simulink model "quarter_sus_imp"  (R2025a)
settings: Solver=FixedStepAuto  StartTime=0.0  StopTime=20  FixedStep=0.001  RelTol=1e-3
model workspace (MAT data in the model file):
  Cs = Simulink.Parameter
  Cs.Value = 2000
  Cs.Complexity = 'real'
  Cs.Dimensions = [1 1]
  Cs.DataType = 'auto'
  Cy_f1 = 128915.5
  Cy_r1 = 85943.6
  G0 = Simulink.Parameter
  G0.Value = 0.000256
  G0.Complexity = 'real'
  G0.Dimensions = [1 1]
  G0.DataType = 'auto'
  IDA_ISD_PBC_bd = Simulink.Parameter
  IDA_ISD_PBC_bd.Value = 300
  IDA_ISD_PBC_bd.Complexity = 'real'
  IDA_ISD_PBC_bd.Dimensions = [1 1]
  IDA_ISD_PBC_bd.DataType = 'auto'
  IDA_ISD_PBC_c1 = Simulink.Parameter
  IDA_ISD_PBC_c1.Value = 1500
  IDA_ISD_PBC_c1.Complexity = 'real'
  IDA_ISD_PBC_c1.Dimensions = [1 1]
  IDA_ISD_PBC_c1.DataType = 'auto'
  IDA_ISD_PBC_k1 = Simulink.Parameter
  IDA_ISD_PBC_k1.Value = 10000
  IDA_ISD_PBC_k1.Complexity = 'real'
  IDA_ISD_PBC_k1.Dimensions = [1 1]
  IDA_ISD_PBC_k1.DataType = 'auto'
  IDA_ISD_PBC_k2 = Simulink.Parameter
  IDA_ISD_PBC_k2.Value = 5000
  IDA_ISD_PBC_k2.Complexity = 'real'
  IDA_ISD_PBC_k2.Dimensions = [1 1]
  IDA_ISD_PBC_k2.DataType = 'auto'
  IDA_ISD_PBC_r1 = Simulink.Parameter
  IDA_ISD_PBC_r1.Value = 1
  IDA_ISD_PBC_r1.Complexity = 'real'
  IDA_ISD_PBC_r1.Dimensions = [1 1]
  IDA_ISD_PBC_r1.DataType = 'auto'
  IDA_PBC_cd4 = 2000
  IDA_PBC_kd2 = 10000
  IDA_PBC_r1 = 1.5
  IDA_PBC_r2 = 0.44
  ISD_1_b = Simulink.Parameter
  ISD_1_b.Value = 158
  ISD_1_b.Complexity = 'real'
  ISD_1_b.Dimensions = [1 1]
  ISD_1_b.DataType = 'auto'
  ISD_1_c = Simulink.Parameter
  ISD_1_c.Value = 500
  ISD_1_c.Complexity = 'real'
  ISD_1_c.Dimensions = [1 1]
  ISD_1_c.DataType = 'auto'
  ISD_1_k1 = Simulink.Parameter
  ISD_1_k1.Value = 1000
  ISD_1_k1.Complexity = 'real'
  ISD_1_k1.Dimensions = [1 1]
  ISD_1_k1.DataType = 'auto'
  ISD_1_k2 = Simulink.Parameter
  ISD_1_k2.Value = 1000
  ISD_1_k2.Complexity = 'real'
  ISD_1_k2.Dimensions = [1 1]
  ISD_1_k2.DataType = 'auto'
  Izz1 = 1536.7
  Ks = Simulink.Parameter
  Ks.Value = 20000
  Ks.Complexity = 'real'
  Ks.Dimensions = [1 1]
  Ks.DataType = 'auto'
  Kt = Simulink.Parameter
  Kt.Value = 200000
  Kt.Complexity = 'real'
  Kt.Dimensions = [1 1]
  Kt.DataType = 'auto'
  Q = Simulink.Parameter
  Q.Value = [0.1  0  0  0; 0  0.1  0  0; 0  0  1  0; 0  0  0  0.1]
  Q.Complexity = 'real'
  Q.Dimensions = [4 4]
  Q.DataType = 'auto'
  Q_dot = Simulink.Parameter
  Q_dot.Value = [1  0; 0  0.001]
  Q_dot.Complexity = 'real'
  Q_dot.Dimensions = [2 2]
  Q_dot.DataType = 'auto'
  Q_dot_s = Simulink.Parameter
  Q_dot_s.Value = 1
  Q_dot_s.Complexity = 'real'
  Q_dot_s.Dimensions = [1 1]
  Q_dot_s.DataType = 'auto'
  Q_dot_u = Simulink.Parameter
  Q_dot_u.Value = 0.001
  Q_dot_u.Complexity = 'real'
  Q_dot_u.Dimensions = [1 1]
  Q_dot_u.DataType = 'auto'
  Q_flec = Simulink.Parameter
  Q_flec.Value = 2.5
  Q_flec.Complexity = 'real'
  Q_flec.Dimensions = [1 1]
  Q_flec.DataType = 'auto'
  SHADD_alpha = Simulink.Parameter
  SHADD_alpha.Value = 11.9
  SHADD_alpha.Complexity = 'real'
  SHADD_alpha.Dimensions = [1 1]
  SHADD_alpha.DataType = 'auto'
  a1 = 1.015
  a_max = Simulink.Parameter
  a_max.Value = 4000
  a_max.Complexity = 'real'
  a_max.Dimensions = [1 1]
  a_max.DataType = 'auto'
  a_min = Simulink.Parameter
  a_min.Value = -4000
  a_min.Complexity = 'real'
  a_min.Dimensions = [1 1]
  a_min.DataType = 'auto'
  adva_max = Simulink.Parameter
  adva_max.Value = 300
  adva_max.Complexity = 'real'
  adva_max.Dimensions = [1 1]
  adva_max.DataType = 'auto'
  adva_min = Simulink.Parameter
  adva_min.Value = -300
  adva_min.Complexity = 'real'
  adva_min.Dimensions = [1 1]
  adva_min.DataType = 'auto'
  as_max = Simulink.Parameter
  as_max.Value = 2
  as_max.Complexity = 'real'
  as_max.Dimensions = [1 1]
  as_max.DataType = 'auto'
  b1 = 1.895
  b_deflec = Simulink.Parameter
  b_deflec.Value = 0.04
  b_deflec.Complexity = 'real'
  b_deflec.Dimensions = [1 1]
  b_deflec.DataType = 'auto'
  b_deflec.DocUnits = 'm'
  bump_height = Simulink.Parameter
  bump_height.Value = 0.02
  bump_height.Complexity = 'real'
  bump_height.Dimensions = [1 1]
  bump_height.DataType = 'auto'
  bump_lenth = Simulink.Parameter
  bump_lenth.Value = 0.3
  bump_lenth.Complexity = 'real'
  bump_lenth.Dimensions = [1 1]
  bump_lenth.DataType = 'auto'
  bump_start = Simulink.Parameter
  bump_start.Value = 1
  bump_start.Complexity = 'real'
  bump_start.Dimensions = [1 1]
  bump_start.DataType = 'auto'
  damper_param = Simulink.Parameter
  damper_param.Value = [-3991.04201041 6552.27356799 -1014.47680093 15090.2668269 -24778.0492645 8455.72459788 2073.28613088 -842.442698484 15.8288582111 -42.6273340405 228.645778088 77.1011895387 -307.938386665 98.5439708573 7.35255277487 0.432771680092]
  damper_param.Complexity = 'real'
  damper_param.Dimensions = [1 16]
  damper_param.DataType = 'auto'
  deflec_max = Simulink.Parameter
  deflec_max.Value = 0.02
  deflec_max.Complexity = 'real'
  deflec_max.Dimensions = [1 1]
  deflec_max.DataType = 'auto'
  done_range = Simulink.Parameter
  done_range.Value = [6 5 0.523598775598]
  done_range.Complexity = 'real'
  done_range.Dimensions = [1 3]
  done_range.DataType = 'double'
  f0 = Simulink.Parameter
  f0.Value = 0.1
  f0.Complexity = 'real'
  f0.Dimensions = [1 1]
  f0.DataType = 'auto'
  h1 = 0.54
  imp_Cs = Simulink.Parameter
  imp_Cs.Value = 1800
  imp_Cs.Complexity = 'real'
  imp_Cs.Dimensions = [1 1]
  imp_Cs.DataType = 'auto'
  imp_Ks = Simulink.Parameter
  imp_Ks.Value = 20500
  imp_Ks.Complexity = 'real'
  imp_Ks.Dimensions = [1 1]
  imp_Ks.DataType = 'auto'
  imp_Ms = Simulink.Parameter
  imp_Ms.Value = 370
  imp_Ms.Complexity = 'real'
  imp_Ms.Dimensions = [1 1]
  imp_Ms.DataType = 'auto'
  inerter_b = Simulink.Parameter
  inerter_b.Value = 300
  inerter_b.Complexity = 'real'
  inerter_b.Dimensions = [1 1]
  inerter_b.DataType = 'auto'
  inerter_b_2 = Simulink.Parameter
  inerter_b_2.Value = 2
  inerter_b_2.Complexity = 'real'
  inerter_b_2.Dimensions = [1 1]
  inerter_b_2.DataType = 'auto'
  inerter_c = Simulink.Parameter
  inerter_c.Value = 2000
  inerter_c.Complexity = 'real'
  inerter_c.Dimensions = [1 1]
  inerter_c.DataType = 'auto'
  inerter_k = Simulink.Parameter
  inerter_k.Value = 5000
  inerter_k.Complexity = 'real'
  inerter_k.Dimensions = [1 1]
  inerter_k.DataType = 'auto'
  inerter_k_2 = Simulink.Parameter
  inerter_k_2.Value = 10000
  inerter_k_2.Complexity = 'real'
  inerter_k_2.Dimensions = [1 1]
  inerter_k_2.DataType = 'auto'
  ms = Simulink.Parameter
  ms.Value = 400
  ms.Complexity = 'real'
  ms.Dimensions = [1 1]
  ms.DataType = 'auto'
  mu = Simulink.Parameter
  mu.Value = 40
  mu.Complexity = 'real'
  mu.Dimensions = [1 1]
  mu.DataType = 'auto'
  noise_seed = Simulink.Parameter
  noise_seed.Value = 23341
  noise_seed.Complexity = 'real'
  noise_seed.Dimensions = [1 1]
  noise_seed.DataType = 'auto'
  punish_Q = Simulink.Parameter
  punish_Q.Value = [10 0.1 1]
  punish_Q.Complexity = 'real'
  punish_Q.Dimensions = [1 3]
  punish_Q.DataType = 'auto'
  punish_R = Simulink.Parameter
  punish_R.Value = 0
  punish_R.Complexity = 'real'
  punish_R.Dimensions = [1 1]
  punish_R.DataType = 'auto'
  reward_w_as = Simulink.Parameter
  reward_w_as.Value = 2
  reward_w_as.Complexity = 'real'
  reward_w_as.Dimensions = [1 1]
  reward_w_as.DataType = 'auto'
  reward_w_au = Simulink.Parameter
  reward_w_au.Value = 40
  reward_w_au.Complexity = 'real'
  reward_w_au.Dimensions = [1 1]
  reward_w_au.DataType = 'auto'
  reward_w_defv = Simulink.Parameter
  reward_w_defv.Value = 0.6
  reward_w_defv.Complexity = 'real'
  reward_w_defv.Dimensions = [1 1]
  reward_w_defv.DataType = 'auto'
  road_seed = Simulink.Parameter
  road_seed.Value = 9759
  road_seed.Complexity = 'real'
  road_seed.Dimensions = [1 1]
  road_seed.DataType = 'auto'
  road_type = Simulink.Parameter
  road_type.Value = 3
  road_type.Complexity = 'real'
  road_type.Dimensions = [1 1]
  road_type.DataType = 'int8'
  sigma_f1 = 0.1
  sigma_r1 = 0.1
  sine_amp = Simulink.Parameter
  sine_amp.Value = 0.01
  sine_amp.Complexity = 'real'
  sine_amp.Dimensions = [1 1]
  sine_amp.DataType = 'auto'
  sine_amp.DocUnits = 'm'
  sine_freq = Simulink.Parameter
  sine_freq.Value = 4
  sine_freq.Complexity = 'real'
  sine_freq.Dimensions = [1 1]
  sine_freq.DataType = 'auto'
  sine_freq.DocUnits = 'Hz'
  u = Simulink.Parameter
  u.Value = 22.2222
  u.Complexity = 'real'
  u.Dimensions = [1 1]
  u.DataType = 'auto'
  vs0 = Simulink.Parameter
  vs0.Value = 0
  vs0.Complexity = 'real'
  vs0.Dimensions = [1 1]
  vs0.DataType = 'auto'
  vu0 = Simulink.Parameter
  vu0.Value = 0
  vu0.Complexity = 'real'
  vu0.Dimensions = [1 1]
  vu0.DataType = 'auto'
  x_max = Simulink.Parameter
  x_max.Value = [9999 9999 9999 9999 9999 9999 9999 9999 9999 9999 9999 9999]
  x_max.Complexity = 'real'
  x_max.Dimensions = [1 12]
  x_max.DataType = 'auto'
  x_min = Simulink.Parameter
  x_min.Value = [-9999 -9999 -9999 -9999 -9999 -9999 -9999 -9999 -9999 -9999 -9999 9999]
  x_min.Complexity = 'real'
  x_min.Dimensions = [1 12]
  x_min.DataType = 'auto'
  xs0 = Simulink.Parameter
  xs0.Value = 0
  xs0.Complexity = 'real'
  xs0.Dimensions = [1 1]
  xs0.DataType = 'auto'
  xu0 = Simulink.Parameter
  xu0.Value = 0
  xu0.Complexity = 'real'
  xu0.Dimensions = [1 1]
  xu0.DataType = 'auto'
undefined symbols (not defined in the file or in its folder): ADD, Force, IDA, Imp, PBC, SH, Train, Validation
libraries: fl_lib x32, nesl_utility x27, sdl_lib x2, deeplib x1, simulink x1
(part 1 of 5)
settings Model: PauseTimes=3  TunableVars=a_max,a_min,adva_max,adva_min,x_ini,x_max,x_min  TunableVarsStorageClass=Auto,Auto,Auto,Auto,Auto,Auto,Auto  TunableVarsTypeQualifier=,,,,,,  ParameterArgumentNames=Cs,G0,Ks,Kt,Q,Q_dot,Q_dot_s,Q_dot_u,Q_flec,a_max,a_min,adva_max,adva_min,as_max,b_deflec,bump_height,bump_lenth,bump_start,damper_param,deflec_max,done_range,f0,inerter_b,inerter_b_2,inerter_c,inerter_k,inerter_k_2,ms,mu,noise_seed,punish_Q,punish_R,road_seed,road_type,sine_amp,sine_freq,u,vs0,vu0,x_max,x_min,xs0,xu0  Creator=hjzsj  LastModifiedBy=Asus
settings ConfigSet: Description=Config for code generation python binding.
settings OptimizationCC: DefaultParameterBehavior=Inlined  UseDivisionForNetSlopeComputation=on  UseFloatMulNetSlope=on  StrengthReduction=on  PassReuseOutputArgsAs=Individual arguments  ZeroExternalMemoryAtStartup=off  ZeroInternalMemoryAtStartup=off  NoFixptDivByZeroProtection=on  EfficientFloat2IntCast=on  OptimizeBlockOrder=speed  OptimizationPriority=Speed  OptimizationCustomize=off  MultiThreadedLoops=on  AutoScheduleForLoops=on  EfficientTunableParamExpr=on
settings DebuggingCC: ParameterTunabilityLossMsg=error  UnconnectedInputMsg=warning  UnconnectedOutputMsg=warning  UnconnectedLineMsg=warning  ArithmeticOperatorsInVariantConditions=warning
settings HardwareCC: ProdLongLongMode=on  TargetPreprocMaxBitsSint=64.0  TargetPreprocMaxBitsUint=64.0
settings ModelReferenceCC: EnableRefExpFcnMdlSchedulingChecks=on
settings SFSimCC: MATLABDynamicMemAlloc=off  CustomCodeUndefinedFunction=UseInterfaceOnly  SimTargetLang=C++  SimDLTargetLibrary=mkl-dnn
settings RTWCC: SystemTargetFile=ert.tlc  GenCodeOnly=on  TemplateMakefile=ert_default_tmf  PostCodeGenCommand=slxpy.postprocess(modelName,buildInfo)  RetainRTWFile=on  Toolchain=MinGW64 | gmake (64-bit Windows)  BuildConfiguration=Debug  PortableWordSizes=on  TargetLang=C++  GPUComputeCapability=3.5  DLArmComputeVersion=19.05  Description=Embedded Coder
settings CodeAppCC: ForceParamTrailComments=on  CommentStyle=Multi-line  IgnoreCustomStorageClasses=off  MaxIdLength=64.0  OperatorAnnotations=on  SimulinkDataObjDesc=on  SFDataObjDesc=on  MATLABFcnDesc=on  MangleLength=4.0  InsertBlockDesc=on  StateflowObjectComments=on  MATLABSourceComments=on
settings ERTTargetCC: ExtModeTransport=0.0  ExtModeStaticAlloc=off  ExtModeMexFile=ext_comm  ExtModeIntrfLevel=Level1  RootIOFormat=Structure reference  ERTCustomFileTemplate=example_file_process.tlc  TargetLangStandard=C++11 (ISO)  CodeInterfacePackaging=C++ class  SubcomponentCodeInterfacePackaging=C++ class  SupportComplex=off  SupportContinuousTime=on  SupportVariableSizeSignals=on

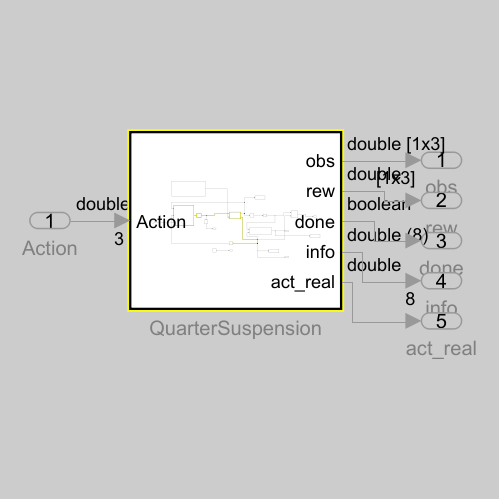
[thumbnail: Simulink's stored preview of the top-level diagram]
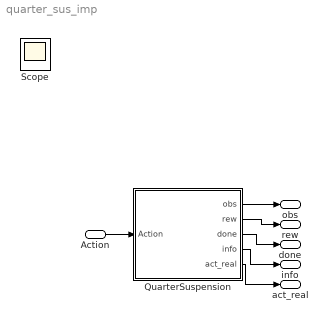
== system quarter_sus_imp ==
  Action : Inport  PortDimensions=3
  "QuarterSuspension " : Subsystem
  obs : Outport
  rew : Outport  Port=2
  done : Outport  Port=3
  info : Outport  Port=4
  act_real : Outport  Port=5
  Scope : Scope
      settings: ActiveDisplayYMinimum=-0.0848  ActiveDisplayYMaximum=0.15745
  wires:
  "QuarterSuspension "/1(obs) -> obs/1
  "QuarterSuspension "/2(rew) -> rew/1
  Action/1 -> "QuarterSuspension "/1(Action)
  "QuarterSuspension "/3(done) -> done/1
  "QuarterSuspension "/4(info) -> info/1
  "QuarterSuspension "/5(act_real) -> act_real/1

== system quarter_sus_imp/QuarterSuspension  ==
  Action : Inport
  Constant : Constant  Value=0  OutDataTypeStr=boolean
  Memory : Memory
  Reshape : Reshape  OutputDimensionality=Row vector (2-D)
  Saturation2 : Saturate  UpperLimit=a_max  LowerLimit=a_min
  Subsystem1 : Subsystem  Variant=on  VariantControlMode=label  VariantControl=Choice  LabelModeActiveChoice=Semi-active Air
  To Workspace : ToWorkspace  VariableName=state  SampleTime=-1
  To Workspace1 : ToWorkspace  VariableName=reward  SampleTime=-1
  To Workspace2 : ToWorkspace  VariableName=info  SampleTime=-1
  Variant Subsystem : Subsystem  Variant=on  VariantControlMode=label  LabelModeActiveChoice=Train-Imp
  Zero-Order Hold : ZeroOrderHold  SampleTime=-1
  Zero-Order Hold2 : ZeroOrderHold  SampleTime=-1
  obs_route : Subsystem
  reward_cal : Subsystem
  road_profile : Subsystem  Variant=on  VariantControlMode=label  LabelModeActiveChoice=OriginRoad
  obs : Outport
  rew : Outport  Port=2
  done : Outport  Port=3
  info : Outport  Port=4
  act_real : Outport  Port=5
  wires:
  Action/1 -> Variant Subsystem/3(train_action)
  Zero-Order Hold/1 -> Reshape/1
  Reshape/1 -> reward_cal/1(state), obs_route/1(state)
  Subsystem1/2(info) -> reward_cal/2(info), To Workspace2/1, info/1, Memory/1, obs_route/2(In3)
  Constant/1 -> done/1
  Variant Subsystem/1(action) -> Saturation2/1
  Saturation2/1 -> Zero-Order Hold2/1, Subsystem1/1(act)
  Zero-Order Hold2/1 -> act_real/1
  road_profile/1("Road ") -> Subsystem1/2(xr)
  Subsystem1/1(state) -> Variant Subsystem/1(state), To Workspace/1, Zero-Order Hold/1
  obs_route/1(obs_out) -> obs/1
  reward_cal/1(reward) -> rew/1, To Workspace1/1
  Memory/1 -> Variant Subsystem/2(ref_info)

== system quarter_sus_imp/QuarterSuspension /Subsystem1 ==
  act : Inport
  xr : Inport  Port=2
  Active Suspension : Subsystem  VariantControl=Active
  Semi Active Air Suspension : Subsystem  VariantControl=Semi-active Air
  Semi Active Air Suspension simscape : Subsystem  VariantControl=Semi-active Air Simscape
  Semi Active Suspension : Subsystem  VariantControl=Semi-active
  state : Outport
  info : Outport  Port=2

== system quarter_sus_imp/QuarterSuspension /Variant Subsystem ==
  note: 1) Add Subsystem or Model blocks as valid variant choices.
      | 2) You cannot connect blocks at this level. At simulation, connectivity is automatically
      | determined, based on the active variant and port name matching.
  state : Inport
  ref_info : Inport  Port=2
  train_action : Inport  Port=3  PortDimensions=3
  ADD : Subsystem  VariantControl=ADD
  H1_power_min : Subsystem  VariantControl=H1_Power_min
  IDA-PBC : Subsystem  VariantControl=IDA-PBC
  Openloop : Subsystem  VariantControl=Opneloop
  PDD : Subsystem  VariantControl=PDD
  SH-ADD : Subsystem  VariantControl=SH-ADD
  Skyhook : Subsystem  VariantControl=SkyHook
  Train-Force : Subsystem  VariantControl=Train-Force
  Train-Imp : Subsystem  VariantControl=Train-Imp
  Vaildation-3para-feedback : Subsystem  VariantControl=Validation-3para-back
  Vaildation-Force : Subsystem  VariantControl=Validation-Force
  Vaildation-Imp : Subsystem  VariantControl=Validation-Imp
  impedance : Subsystem  VariantControl=Impedance
  train_IMP_force : Subsystem  VariantControl=Subsystem
  action : Outport

== system quarter_sus_imp/QuarterSuspension /obs_route ==
  state : Inport
  In3 : Inport  Port=2
  Add : Sum  Inputs=+-
  Reshape : Reshape  OutputDimensionality=Row vector (2-D)
  Selector : Selector  InputPortWidth=8  IndexOptions=Index vector (dialog)  Indices=[7 8]  OutputSizes=1
  Selector1 : Selector  InputPortWidth=4  IndexOptions=Index vector (dialog)  Indices=[1]  OutputSizes=1
  Selector2 : Selector  InputPortWidth=4  IndexOptions=Index vector (dialog)  Indices=[3]  OutputSizes=1
  Vector Concatenate : Concatenate
  obs_out : Outport
  wires:
  Selector/1 -> Vector Concatenate/2
  Selector2/1 -> Add/2
  In3/1 -> Selector/1
  state/1 -> Selector2/1, Selector1/1
  Vector Concatenate/1 -> Reshape/1
  Selector1/1 -> Add/1
  Add/1 -> Vector Concatenate/1
  Reshape/1 -> obs_out/1

== system quarter_sus_imp/QuarterSuspension /reward_cal ==
  state : Inport
  info : Inport  Port=2
  Add : Sum
  Add1 : Sum  Inputs=+-
  Add2 : Sum
  Constant1 : Constant  Value=Q_flec
  Constant3 : Constant  Value=b_deflec
  Demux : Demux  Outputs=2
  Gain : Gain  Gain=Q_dot_s
  Gain1 : Gain  Gain=Q_dot_u
  Gain2 : Gain  Gain=-1
  Selector : Selector  InputPortWidth=8  IndexOptions=Index vector (dialog)  Indices=[7 8]  OutputSizes=1
  Selector1 : Selector  InputPortWidth=4  IndexOptions=Index vector (dialog)  Indices=[1]  OutputSizes=1
  Selector2 : Selector  InputPortWidth=4  IndexOptions=Index vector (dialog)  Indices=[3]  OutputSizes=1
  Square : Math  Operator=square
  Square1 : Math  Operator=square
  cal_reward : MATLAB Function  TreatAsAtomicUnit=on
  reward : Outport
  wires:
  Constant1/1 -> cal_reward/3(Q_flec)
  Constant3/1 -> cal_reward/2(b_def)
  cal_reward/1(reward) -> Add/1  "reward_deflec"
  Add/1 -> Gain2/1  "reward"
  Add2/1 -> Add/2  "reward_dot"
  state/1 -> Selector2/1, Selector1/1
  Selector2/1 -> Add1/2
  Selector1/1 -> Add1/1
  Add1/1 -> cal_reward/1(state_deflec)
  info/1 -> Selector/1
  Selector/1 -> Demux/1
  Demux/1 -> Square/1
  Demux/2 -> Square1/1
  Square/1 -> Gain/1
  Square1/1 -> Gain1/1
  Gain2/1 -> reward/1
  Gain/1 -> Add2/1  "reward_accs"
  Gain1/1 -> Add2/2  "reward_accu"

== system quarter_sus_imp/QuarterSuspension /road_profile ==
  note: 1) Add Subsystem or Model blocks as valid variant choices.
      | 2) You cannot connect blocks at this level. At simulation, connectivity is automatically
      | determined, based on the active variant and port name matching.
  Subsystem : Subsystem  VariantControl=Look table
  gp : Subsystem  VariantControl=GpSample
  origin : Subsystem  VariantControl=OriginRoad
  "Road " : Outport

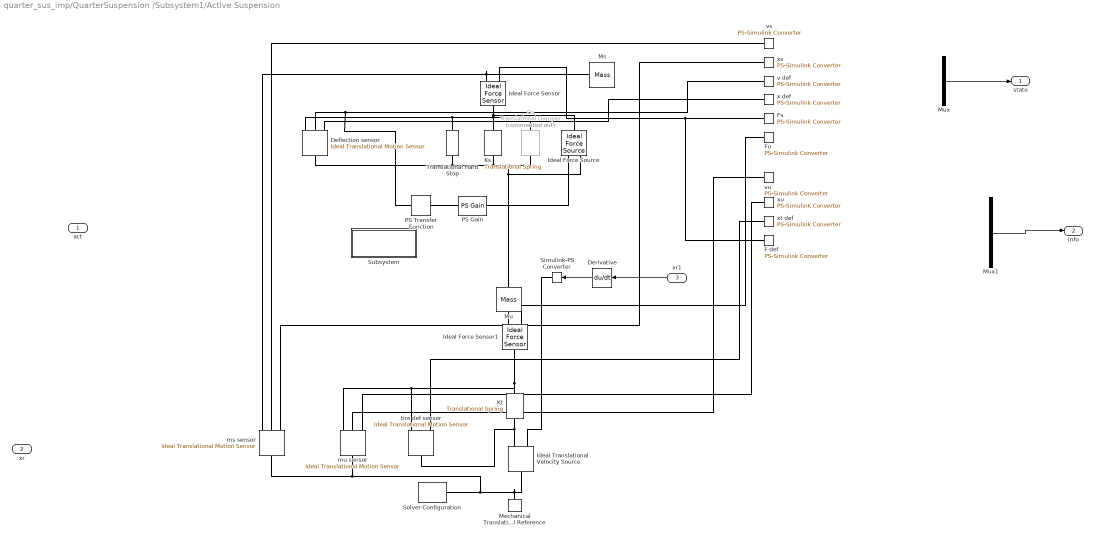
== system quarter_sus_imp/QuarterSuspension /Subsystem1/Active Suspension ==
  act : Inport
  xr : Inport  Port=2
  xr1 : Inport  Port=3
  Cs : fl_lib/Mechanical/Translational Elements/Translational Damper  Commented=on  D=2000 N*s/m  v_specify=on  v_priority=None  v=0 m/s  v_nominal_specify=off  v_nominal_unit=m/s  v_nominal_value=1  f_specify=off  f_priority=None  f=0 N  f_nominal_specify=off  f_nominal_unit=N  f_nominal_value=1
  Deflection sensor : fl_lib/Mechanical/Mechanical Sensors/Ideal Translational Motion Sensor  reference=foundation.enum.MeasurementReference.difference  acceleration_port=false  velocity_port=true  position_port=true  offset=0 m
  Derivative : Derivative
  F def : nesl_utility/PS-Simulink Converter  PhysicalDomain=network_engine_domain  SubClassName=ps_output  LeftPortType=input  RightPortType=output  PseudoPeriodic=off  Frequencies=[]  VectorFormat=inherit  Unit=inherit  AffineConversion=off
  Fs : nesl_utility/PS-Simulink Converter  PhysicalDomain=network_engine_domain  SubClassName=ps_output  LeftPortType=input  RightPortType=output  PseudoPeriodic=off  Frequencies=[]  VectorFormat=inherit  Unit=inherit  AffineConversion=off
  Fu : nesl_utility/PS-Simulink Converter  PhysicalDomain=network_engine_domain  SubClassName=ps_output  LeftPortType=input  RightPortType=output  PseudoPeriodic=off  Frequencies=[]  VectorFormat=inherit  Unit=inherit  AffineConversion=off
  Ideal Force Sensor : fl_lib/Mechanical/Mechanical Sensors/Ideal Force Sensor
  Ideal Force Sensor1 : fl_lib/Mechanical/Mechanical Sensors/Ideal Force Sensor
  Ideal Force Source : fl_lib/Mechanical/Mechanical Sources/Ideal Force Source
      settings: LogSimulationData=on
  Ideal Translational Velocity Source : fl_lib/Mechanical/Mechanical Sources/Ideal Translational Velocity Source
  Ks : fl_lib/Mechanical/Translational Elements/Translational Spring  spr_rate=20000 N/m  v_specify=off  v_priority=None  v=0 m/s  v_nominal_specify=off  v_nominal_unit=m/s  v_nominal_value=1  f_specify=off  f_priority=None  f=0 N  f_nominal_specify=off  f_nominal_unit=N  f_nominal_value=1  x_specify=on  x_priority=High  x=0 m  x_nominal_specify=off  x_nominal_unit=m  x_nominal_value=1
  Kt : fl_lib/Mechanical/Translational Elements/Translational Spring  spr_rate=200000 N/m  v_specify=off  v_priority=None  v=0 m/s  v_nominal_specify=off  v_nominal_unit=m/s  v_nominal_value=1  f_specify=off  f_priority=None  f=0 N  f_nominal_specify=off  f_nominal_unit=N  f_nominal_value=1  x_specify=on  x_priority=High  x=0 m  x_nominal_specify=off  x_nominal_unit=m  x_nominal_value=1
  Mechanical Translational Reference : fl_lib/Mechanical/Translational Elements/Mechanical Translational Reference
  Ms : fl_lib/Mechanical/Translational Elements/Mass  mass=400 kg  num_ports=foundation.enum.numPorts2.one  v_specify=off  v_priority=High  v=0 m/s  v_nominal_specify=off  v_nominal_unit=m/s  v_nominal_value=1  f_specify=off  f_priority=None  f=0 N  f_nominal_specify=off  f_nominal_unit=N  f_nominal_value=1
  Mu : fl_lib/Mechanical/Translational Elements/Mass  mass=40 kg  num_ports=foundation.enum.numPorts2.two  v_specify=off  v_priority=High  v=0 m/s  v_nominal_specify=off  v_nominal_unit=m/s  v_nominal_value=1  f_specify=off  f_priority=None  f=0 N  f_nominal_specify=off  f_nominal_unit=N  f_nominal_value=1
      settings: InternalSimscapePortConfiguration="{\"Bottom\":[],\"Left\":[{\"id\":\"M\",\"label\":\"\",\"type\":\"foundation.mechanical.translational.translational\"}],\"Right\":[{\"id\":\"N\",\"label\":\"\",\"type\":\"foundation.mechanical.translational.translational\"}],\"Top\":[]}"
  Mux : Mux
  Mux1 : Mux  Inputs=8
  PS Gain : fl_lib/Physical Signals/Functions/PS Gain  gain=2000 N*s/m
  PS Transfer Function : fl_lib/Physical Signals/Linear Operators/PS Transfer Function  transfer_function_type=foundation.enum.transfer_function_type.lag  T=20 ms  T1=2 s  T2=1 s  reset_method=foundation.enum.IntegratorResetSpec.None  initial_condition_spec=foundation.enum.IntegratorICSpec.Internal  y0=0 m/s
      settings: InternalSimscapePortConfiguration="{\"Bottom\":[],\"Left\":[{\"id\":\"U\",\"label\":\"\",\"type\":\"input\"}],\"Right\":[{\"id\":\"Y\",\"label\":\"\",\"type\":\"output\"}],\"Top\":[]}"
  Simulink-PS Converter : nesl_utility/Simulink-PS Converter  PhysicalDomain=network_engine_domain  SubClassName=ps_input  LeftPortType=input  RightPortType=output  PseudoPeriodic=off  Frequencies=[]  NoiseDistribution=none  NoiseParameters=[]  Unit=1  AffineConversion=off  FilteringAndDerivatives=provide  SimscapeFilterOrder=1  InputFilterTimeConstant=0.001  UdotUserProvided=0
  Solver Configuration : nesl_utility/Solver Configuration  PhysicalDomain=network_engine_domain  SubClassName=solver  LeftPortType=input  RightPortType=generic  Tones=[]  Harmonics=[]  SimulateNoise=off  Profile=off  UseLocalSampling=off  EnableSwitchedLinearOptims=on  FrequencyDomain=off  UseCCode=off  RelTol=0.001  AbsTol=1e-06  MinStep=1e-09  ToWorkspace=off  RevertToSquareIcSolve=off  NumHomotopyIterations=100  PhasorMode=off  PhasorModeNumHarmonics=1  ConsistencySolver=NEWTON_XTOL_AFTER_FTOL  IndexReductionMethod=DerivativeReplacement  DoDC=off  ResidualTolerance=1e-09  ConsistencyTolSource=GLOBAL  ConsistencyAbsTol=0.001  ConsistencyRelTol=0.001  ConsistencyTolFactor=0.001  UseLocalSolver=off  LocalSolverChoice=NE_BACKWARD_EULER_ADVANCER  ResolveIndetEquations=on  FunctionEvalNumThread=1  LocalSolverSampleTime=0.001  DoFixedCost=off  MaxNonlinIter=3  MaxModeIter=2  ComputeImpulses=off  ImpulseIterations=2  LinearAlgebra=auto  LinearAlgebraNumThread=0  EquationFormulation=NE_TIME_EF  DelaysMemoryBudget=1024  AutomaticFiltering=on  FilteringTimeConstant=0.001  PartitionStorageMethod=AS_NEEDED  PartitionMemoryBudget=1024  PartitionMethod=ROBUST
  Subsystem : Subsystem
  Translational Hard Stop : fl_lib/Mechanical/Translational Elements/Translational Hard Stop  upper_bnd=0.2 m  lower_bnd=-0.2 m  model=simscape.enum.hardstop.smooth  stiff_up=1e6 N/m  stiff_low=1e6 N/m  D_up=150 N*s/m  D_low=150 N*s/m  transition=0.01 mm  coeff_rest=0.7  v_tol=0.001 m/s  f_tol=0.001 N  x_specify=on  x_priority=High  x=0 m  x_nominal_specify=off  x_nominal_unit=m  x_nominal_value=1  v_specify=off  v_priority=None  v=0 m/s  v_nominal_specify=off  v_nominal_unit=m/s  v_nominal_value=1  f_specify=off  f_priority=None  f=0 N  f_nominal_specify=off  f_nominal_unit=N  f_nominal_value=1  M_specify=off  M_priority=None  M=0
  ms sensor : fl_lib/Mechanical/Mechanical Sensors/Ideal Translational Motion Sensor  reference=foundation.enum.MeasurementReference.difference  acceleration_port=false  velocity_port=true  position_port=true  offset=0 m
  mu sensor : fl_lib/Mechanical/Mechanical Sensors/Ideal Translational Motion Sensor  reference=foundation.enum.MeasurementReference.difference  acceleration_port=false  velocity_port=true  position_port=true  offset=0 m
  tire def sensor : fl_lib/Mechanical/Mechanical Sensors/Ideal Translational Motion Sensor  reference=foundation.enum.MeasurementReference.difference  acceleration_port=false  velocity_port=true  position_port=true  offset=0 m
  v def : nesl_utility/PS-Simulink Converter  PhysicalDomain=network_engine_domain  SubClassName=ps_output  LeftPortType=input  RightPortType=output  PseudoPeriodic=off  Frequencies=[]  VectorFormat=inherit  Unit=inherit  AffineConversion=off
  vs : nesl_utility/PS-Simulink Converter  PhysicalDomain=network_engine_domain  SubClassName=ps_output  LeftPortType=input  RightPortType=output  PseudoPeriodic=off  Frequencies=[]  VectorFormat=inherit  Unit=inherit  AffineConversion=off
  vu : nesl_utility/PS-Simulink Converter  PhysicalDomain=network_engine_domain  SubClassName=ps_output  LeftPortType=input  RightPortType=output  PseudoPeriodic=off  Frequencies=[]  VectorFormat=inherit  Unit=inherit  AffineConversion=off
  x def : nesl_utility/PS-Simulink Converter  PhysicalDomain=network_engine_domain  SubClassName=ps_output  LeftPortType=input  RightPortType=output  PseudoPeriodic=off  Frequencies=[]  VectorFormat=inherit  Unit=inherit  AffineConversion=off
  xs : nesl_utility/PS-Simulink Converter  PhysicalDomain=network_engine_domain  SubClassName=ps_output  LeftPortType=input  RightPortType=output  PseudoPeriodic=off  Frequencies=[]  VectorFormat=inherit  Unit=inherit  AffineConversion=off
  xt def : nesl_utility/PS-Simulink Converter  PhysicalDomain=network_engine_domain  SubClassName=ps_output  LeftPortType=input  RightPortType=output  PseudoPeriodic=off  Frequencies=[]  VectorFormat=inherit  Unit=inherit  AffineConversion=off
  xu : nesl_utility/PS-Simulink Converter  PhysicalDomain=network_engine_domain  SubClassName=ps_output  LeftPortType=input  RightPortType=output  PseudoPeriodic=off  Frequencies=[]  VectorFormat=inherit  Unit=inherit  AffineConversion=off
  state : Outport
  info : Outport  Port=2
  wires:
  Mux1/1 -> info/1
  Mux/1 -> state/1
  xr1/1 -> Derivative/1
  Derivative/1 -> Simulink-PS Converter/1
  connections:
  Ideal Translational Velocity Source/LConn1 -- Mechanical Translational Reference/LConn1 -- Solver Configuration/RConn1 -- ms sensor/LConn1 -- mu sensor/LConn1
  Mu/RConn1 -- Deflection sensor/LConn1 -- Translational Hard Stop/LConn1 -- Ks/LConn1 -- Cs/LConn1 -- Ideal Force Source/RConn2
  Ideal Force Sensor/LConn1 -- Ks/RConn1 -- Translational Hard Stop/RConn1 -- Deflection sensor/RConn1 -- Cs/RConn1 -- Ideal Force Source/LConn1
  tire def sensor/LConn1 -- Ideal Translational Velocity Source/RConn2 -- Kt/LConn1
  Ms/LConn1 -- ms sensor/RConn1 -- Ideal Force Sensor/RConn1
  tire def sensor/RConn1 -- mu sensor/RConn1 -- Kt/RConn1 -- Ideal Force Sensor1/LConn1
  Deflection sensor/RConn2 -- v def/LConn1 -- PS Transfer Function/LConn1
  F def/LConn1 -- Ideal Force Sensor/RConn2 -- Fs/LConn1
  PS Gain/LConn1 -- PS Transfer Function/RConn1
  xs/LConn1 -- ms sensor/RConn3
  Ideal Force Sensor1/RConn2 -- Fu/LConn1
  vs/LConn1 -- ms sensor/RConn2
  tire def sensor/RConn3 -- xt def/LConn1
  Ideal Force Sensor1/RConn1 -- Mu/LConn1
  Simulink-PS Converter/RConn1 -- Ideal Translational Velocity Source/RConn1
  vu/LConn1 -- mu sensor/RConn2
  x def/LConn1 -- Deflection sensor/RConn3
  xu/LConn1 -- mu sensor/RConn3
  PS Gain/RConn1 -- Ideal Force Source/RConn1

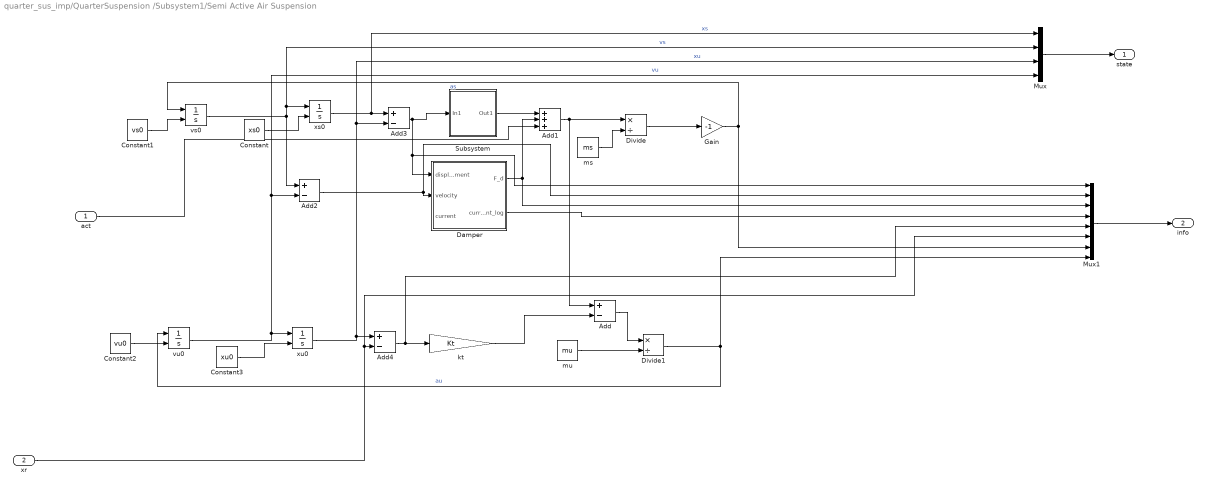
== system quarter_sus_imp/QuarterSuspension /Subsystem1/Semi Active Air Suspension ==
  act : Inport
  xr : Inport  Port=2
  Add{,2..4} (4 alike) : Sum  Inputs=+-
  Add1 : Sum  Inputs=+++
  Constant : Constant  Value=xs0
  Constant1 : Constant  Value=vs0
  Constant2 : Constant  Value=vu0
  Constant3 : Constant  Value=xu0
  Damper : Subsystem  Variant=on  VariantControlMode=label  VariantControl=Choice  LabelModeActiveChoice=simple linear
  Divide : Product  Inputs=*/
  Divide1 : Product  Inputs=*/
  Gain : Gain  Gain=-1
  Mux : Mux
  Mux1 : Mux  Inputs=8
  Subsystem : Subsystem  Variant=on  VariantControlMode=label  LabelModeActiveChoice=linear
  kt : Gain  Gain=Kt
  ms : Constant  Value=ms
  mu : Constant  Value=mu
  vs0 : Integrator  InitialConditionSource=external  InitialCondition=vs0
  vu0 : Integrator  InitialConditionSource=external  InitialCondition=vu0
  xs0 : Integrator  InitialConditionSource=external  InitialCondition=xs0
  xu0 : Integrator  InitialConditionSource=external  InitialCondition=xu0
  state : Outport
  info : Outport  Port=2
  wires:
  Add/1 -> Divide1/1
  Mux1/1 -> info/1
  Mux/1 -> state/1
  act/1 -> Add1/3
  Divide1/1 -> vu0/1, Mux1/8  "au"
  vs0/1 -> xs0/1, Mux/2, Add2/1  "vs"
  Gain/1 -> vs0/1, Mux1/7  "as"
  Damper/2(current_log) -> Mux1/4
  mu/1 -> Divide1/2
  Add4/1 -> Mux1/5, kt/1
  Damper/1(F_d) -> Add1/2, Mux1/3
  ms/1 -> Divide/2
  Add2/1 -> Mux1/2, Damper/2(velocity)
  Add3/1 -> Damper/1(displacement), Mux1/1, Subsystem/1(In1)
  xr/1 -> Add4/2, Mux1/6
  Add1/1 -> Add/1, Divide/1
  xs0/1 -> Add3/1, Mux/1  "xs"
  xu0/1 -> Add4/1, Add3/2, Mux/3  "xu"
  kt/1 -> Add/2
  vu0/1 -> xu0/1, Add2/2, Mux/4  "vu"
  Divide/1 -> Gain/1
  Subsystem/1(Out1) -> Add1/1
  Constant/1 -> xs0/2
  Constant1/1 -> vs0/2
  Constant2/1 -> vu0/2
  Constant3/1 -> xu0/2

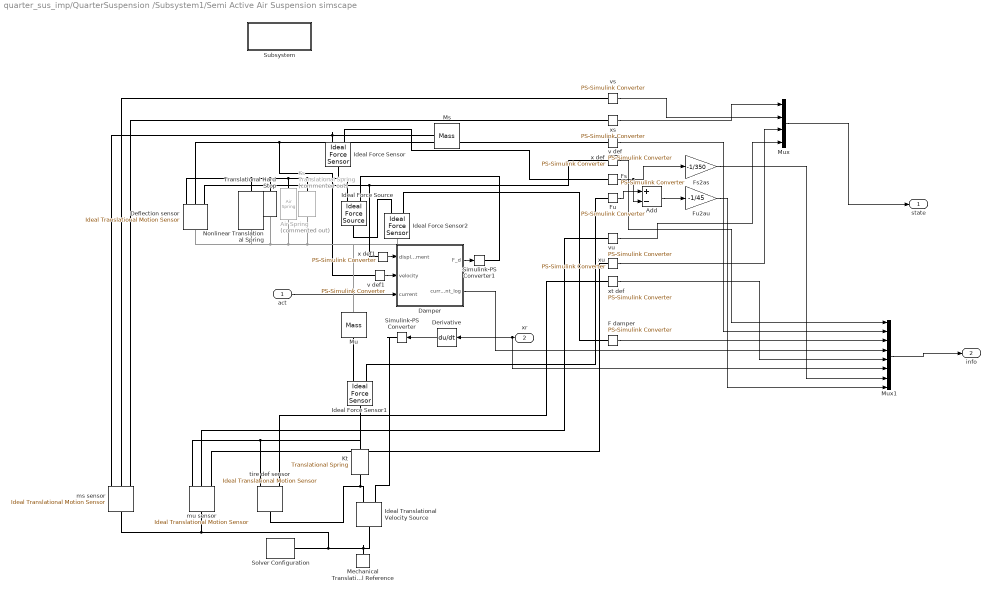
== system quarter_sus_imp/QuarterSuspension /Subsystem1/Semi Active Air Suspension simscape ==
  act : Inport
  xr : Inport  Port=2
  Add : Sum  Inputs=+-
  Air Spring : sdl_lib/Couplings & Drives/Air Spring  Commented=on  parameterization=sdl.enum.AirSpringParameterization.Load  height_vector=[11, 12, 14, 16, 18,20, 22, 24,25] cm  load_vector=[6000, 6200, 6900, 7600, 8400, 9100, 10200, 13000, 18300] N  stiffness_vector=[600, 300, 100, 80, 40, 5] N/cm  damping_vector=[0 0 0 0 0 0 0 0 0 ] N*s/cm  interp_method=simscape.enum.interpolation.smooth  extrap_method=simscape.enum.extrapolation.linear  top_hard_stop=simscape.enum.onoff.off  max_height=25 cm  bottom_hard_stop=simscape.enum.onoff.off  min_height=5 cm  hard_stop_model=simscape.enum.hardstop.smooth  top_stiffness=1e8 N/cm  top_damping=1e8 N*s/cm  bottom_stiffness=1e8 N/cm  bottom_damping=1e8 N*s/cm  transition=0.1 mm  coeff_rest=0.7  v_tol=0.001 m/s  f_tol=0.001 N  height_specify=on  height_priority=High  height=18 cm  height_nominal_specify=off  height_nominal_unit=cm  height_nominal_value=1  v_specify=off  v_priority=None  v=0 m/s  v_nominal_specify=off  v_nominal_unit=m/s  v_nominal_value=1  f_specify=off  f_priority=None  f=1000 N  f_nominal_specify=off  f_nominal_unit=N  f_nominal_value=1
      settings: InternalSimscapePortConfiguration="{\"Bottom\":[],\"Left\":[{\"id\":\"R\",\"label\":\"R\",\"type\":\"foundation.mechanical.translational.translational\"}],\"Right\":[{\"id\":\"C\",\"label\":\"C\",\"type\":\"foundation.mechanical.translational.translational\"}],\"Top\":[]}"
  Damper : Subsystem  Variant=on  VariantControlMode=label  VariantControl=Choice  LabelModeActiveChoice=Semi-active
  Deflection sensor : fl_lib/Mechanical/Mechanical Sensors/Ideal Translational Motion Sensor  reference=foundation.enum.MeasurementReference.difference  acceleration_port=false  velocity_port=true  position_port=true  offset=0 m
      settings: LogSimulationData=on
  Derivative : Derivative
  F damper : nesl_utility/PS-Simulink Converter  PhysicalDomain=network_engine_domain  SubClassName=ps_output  LeftPortType=input  RightPortType=output  PseudoPeriodic=off  Frequencies=[]  VectorFormat=inherit  Unit=inherit  AffineConversion=off
  Fs : nesl_utility/PS-Simulink Converter  PhysicalDomain=network_engine_domain  SubClassName=ps_output  LeftPortType=input  RightPortType=output  PseudoPeriodic=off  Frequencies=[]  VectorFormat=inherit  Unit=inherit  AffineConversion=off
  Fs2as : Gain  Gain=-1/350
  Fu : nesl_utility/PS-Simulink Converter  PhysicalDomain=network_engine_domain  SubClassName=ps_output  LeftPortType=input  RightPortType=output  PseudoPeriodic=off  Frequencies=[]  VectorFormat=inherit  Unit=inherit  AffineConversion=off
  Fu2au : Gain  Gain=-1/45
  Ideal Force Sensor : fl_lib/Mechanical/Mechanical Sensors/Ideal Force Sensor
  Ideal Force Sensor1 : fl_lib/Mechanical/Mechanical Sensors/Ideal Force Sensor
  Ideal Force Sensor2 : fl_lib/Mechanical/Mechanical Sensors/Ideal Force Sensor
  Ideal Force Source : fl_lib/Mechanical/Mechanical Sources/Ideal Force Source
  Ideal Translational Velocity Source : fl_lib/Mechanical/Mechanical Sources/Ideal Translational Velocity Source
  Ks : fl_lib/Mechanical/Translational Elements/Translational Spring  Commented=on  spr_rate=22000 N/m  v_specify=off  v_priority=None  v=0 m/s  v_nominal_specify=off  v_nominal_unit=m/s  v_nominal_value=1  f_specify=off  f_priority=None  f=0 N  f_nominal_specify=off  f_nominal_unit=N  f_nominal_value=1  x_specify=on  x_priority=High  x=0 cm  x_nominal_specify=off  x_nominal_unit=m  x_nominal_value=1
  Kt : fl_lib/Mechanical/Translational Elements/Translational Spring  spr_rate=200000 N/m  v_specify=off  v_priority=None  v=0 m/s  v_nominal_specify=off  v_nominal_unit=m/s  v_nominal_value=1  f_specify=off  f_priority=None  f=0 N  f_nominal_specify=off  f_nominal_unit=N  f_nominal_value=1  x_specify=on  x_priority=High  x=0 m  x_nominal_specify=off  x_nominal_unit=m  x_nominal_value=1
  Mechanical Translational Reference : fl_lib/Mechanical/Translational Elements/Mechanical Translational Reference
  Ms : fl_lib/Mechanical/Translational Elements/Mass  mass=350 kg  num_ports=foundation.enum.numPorts2.one  v_specify=off  v_priority=High  v=0 m/s  v_nominal_specify=off  v_nominal_unit=m/s  v_nominal_value=1  f_specify=off  f_priority=None  f=0 N  f_nominal_specify=off  f_nominal_unit=N  f_nominal_value=1
  Mu : fl_lib/Mechanical/Translational Elements/Mass  mass=45 kg  num_ports=foundation.enum.numPorts2.two  v_specify=off  v_priority=High  v=0 m/s  v_nominal_specify=off  v_nominal_unit=m/s  v_nominal_value=1  f_specify=off  f_priority=None  f=0 N  f_nominal_specify=off  f_nominal_unit=N  f_nominal_value=1
      settings: InternalSimscapePortConfiguration="{\"Bottom\":[],\"Left\":[{\"id\":\"M\",\"label\":\"\",\"type\":\"foundation.mechanical.translational.translational\"}],\"Right\":[{\"id\":\"N\",\"label\":\"\",\"type\":\"foundation.mechanical.translational.translational\"}],\"Top\":[]}"
  Mux : Mux
  Mux1 : Mux  Inputs=8
  Nonlinear Translational Spring : sdl_lib/Couplings & Drives/Springs & Dampers/Nonlinear Translational Spring  parameterization=sdl.enum.polynomialTLU.tlu  symmetry=sdl.enum.symmetry.symmetric  coefficient_vector=[100, 0, 10, 0, 1] N/m  tension_coefficient_vector=[100, 0, 10, 0, 1] N/m  compression_coefficient_vector=[1000, -10, 100, 0, 0] N/m  deformation_vector=[-0.04,-0.03, -0.02, -0.01, -0.005,-0.004, -0.002,-0.001,0.00, 0.001, 0.002,0.004,0.005,0.01, 0.02,0.03, 0.04] m  force_vector=[-1300,-835,-505,-240,-115,-90,-48,-25,0,10,30,60,80,165,320,435,470] N  interp_method=simscape.enum.interpolation.smooth  extrap_method=simscape.enum.extrapolation.linear  x_specify=off  x_priority=High  x=0 m  x_nominal_specify=off  x_nominal_unit=m  x_nominal_value=1
      settings: InternalSimscapePortConfiguration="{\"Bottom\":[],\"Left\":[{\"id\":\"R\",\"label\":\"R\",\"type\":\"foundation.mechanical.translational.translational\"}],\"Right\":[{\"id\":\"C\",\"label\":\"C\",\"type\":\"foundation.mechanical.translational.translational\"}],\"Top\":[]}"
  Simulink-PS Converter : nesl_utility/Simulink-PS Converter  PhysicalDomain=network_engine_domain  SubClassName=ps_input  LeftPortType=input  RightPortType=output  PseudoPeriodic=off  Frequencies=[]  NoiseDistribution=none  NoiseParameters=[]  Unit=1  AffineConversion=off  FilteringAndDerivatives=provide  SimscapeFilterOrder=1  InputFilterTimeConstant=0.001  UdotUserProvided=0
  Simulink-PS Converter1 : nesl_utility/Simulink-PS Converter  PhysicalDomain=network_engine_domain  SubClassName=ps_input  LeftPortType=input  RightPortType=output  PseudoPeriodic=off  Frequencies=[]  NoiseDistribution=none  NoiseParameters=[]  Unit=N  AffineConversion=off  FilteringAndDerivatives=provide  SimscapeFilterOrder=1  InputFilterTimeConstant=0.001  UdotUserProvided=0
  Solver Configuration : nesl_utility/Solver Configuration  PhysicalDomain=network_engine_domain  SubClassName=solver  LeftPortType=input  RightPortType=generic  Tones=[]  Harmonics=[]  SimulateNoise=off  Profile=off  UseLocalSampling=off  EnableSwitchedLinearOptims=on  FrequencyDomain=off  UseCCode=off  RelTol=0.001  AbsTol=1e-06  MinStep=1e-09  ToWorkspace=off  RevertToSquareIcSolve=off  NumHomotopyIterations=100  PhasorMode=off  PhasorModeNumHarmonics=1  ConsistencySolver=NEWTON_XTOL_AFTER_FTOL  IndexReductionMethod=DerivativeReplacement  DoDC=off  ResidualTolerance=1e-09  ConsistencyTolSource=GLOBAL  ConsistencyAbsTol=0.001  ConsistencyRelTol=0.001  ConsistencyTolFactor=0.001  UseLocalSolver=off  LocalSolverChoice=NE_BACKWARD_EULER_ADVANCER  ResolveIndetEquations=on  FunctionEvalNumThread=1  LocalSolverSampleTime=0.001  DoFixedCost=off  MaxNonlinIter=3  MaxModeIter=2  ComputeImpulses=off  ImpulseIterations=2  LinearAlgebra=auto  LinearAlgebraNumThread=0  EquationFormulation=NE_TIME_EF  DelaysMemoryBudget=1024  AutomaticFiltering=on  FilteringTimeConstant=0.001  PartitionStorageMethod=AS_NEEDED  PartitionMemoryBudget=1024  PartitionMethod=ROBUST
  Subsystem : Subsystem
  Translational Hard Stop : fl_lib/Mechanical/Translational Elements/Translational Hard Stop  upper_bnd=4 cm  lower_bnd=-4 cm  model=simscape.enum.hardstop.smooth  stiff_up=1e7 N/m  stiff_low=1e7 N/m  D_up=5000 N*s/m  D_low=5000 N*s/m  transition=0.01 mm  coeff_rest=0.7  v_tol=0.001 m/s  f_tol=0.001 N  x_specify=on  x_priority=High  x=0 cm  x_nominal_specify=off  x_nominal_unit=m  x_nominal_value=1  v_specify=off  v_priority=None  v=0 m/s  v_nominal_specify=off  v_nominal_unit=m/s  v_nominal_value=1  f_specify=off  f_priority=None  f=0 N  f_nominal_specify=off  f_nominal_unit=N  f_nominal_value=1  M_specify=off  M_priority=None  M=0
      settings: LogSimulationData=on
  ms sensor : fl_lib/Mechanical/Mechanical Sensors/Ideal Translational Motion Sensor  reference=foundation.enum.MeasurementReference.difference  acceleration_port=false  velocity_port=true  position_port=true  offset=0 m
  mu sensor : fl_lib/Mechanical/Mechanical Sensors/Ideal Translational Motion Sensor  reference=foundation.enum.MeasurementReference.difference  acceleration_port=false  velocity_port=true  position_port=true  offset=0 m
  tire def sensor : fl_lib/Mechanical/Mechanical Sensors/Ideal Translational Motion Sensor  reference=foundation.enum.MeasurementReference.difference  acceleration_port=false  velocity_port=true  position_port=true  offset=0 m
  v def : nesl_utility/PS-Simulink Converter  PhysicalDomain=network_engine_domain  SubClassName=ps_output  LeftPortType=input  RightPortType=output  PseudoPeriodic=off  Frequencies=[]  VectorFormat=inherit  Unit=inherit  AffineConversion=off
  v def1 : nesl_utility/PS-Simulink Converter  PhysicalDomain=network_engine_domain  SubClassName=ps_output  LeftPortType=input  RightPortType=output  PseudoPeriodic=off  Frequencies=[]  VectorFormat=inherit  Unit=inherit  AffineConversion=off
  vs : nesl_utility/PS-Simulink Converter  PhysicalDomain=network_engine_domain  SubClassName=ps_output  LeftPortType=input  RightPortType=output  PseudoPeriodic=off  Frequencies=[]  VectorFormat=inherit  Unit=inherit  AffineConversion=off
  vu : nesl_utility/PS-Simulink Converter  PhysicalDomain=network_engine_domain  SubClassName=ps_output  LeftPortType=input  RightPortType=output  PseudoPeriodic=off  Frequencies=[]  VectorFormat=inherit  Unit=inherit  AffineConversion=off
  x def : nesl_utility/PS-Simulink Converter  PhysicalDomain=network_engine_domain  SubClassName=ps_output  LeftPortType=input  RightPortType=output  PseudoPeriodic=off  Frequencies=[]  VectorFormat=inherit  Unit=inherit  AffineConversion=off
  x def1 : nesl_utility/PS-Simulink Converter  PhysicalDomain=network_engine_domain  SubClassName=ps_output  LeftPortType=input  RightPortType=output  PseudoPeriodic=off  Frequencies=[]  VectorFormat=inherit  Unit=inherit  AffineConversion=off
  xs : nesl_utility/PS-Simulink Converter  PhysicalDomain=network_engine_domain  SubClassName=ps_output  LeftPortType=input  RightPortType=output  PseudoPeriodic=off  Frequencies=[]  VectorFormat=inherit  Unit=inherit  AffineConversion=off
  xt def : nesl_utility/PS-Simulink Converter  PhysicalDomain=network_engine_domain  SubClassName=ps_output  LeftPortType=input  RightPortType=output  PseudoPeriodic=off  Frequencies=[]  VectorFormat=inherit  Unit=inherit  AffineConversion=off
  xu : nesl_utility/PS-Simulink Converter  PhysicalDomain=network_engine_domain  SubClassName=ps_output  LeftPortType=input  RightPortType=output  PseudoPeriodic=off  Frequencies=[]  VectorFormat=inherit  Unit=inherit  AffineConversion=off
  state : Outport
  info : Outport  Port=2
  wires:
  Mux1/1 -> info/1
  Mux/1 -> state/1
  act/1 -> Damper/3(current)
  v def1/1 -> Damper/2(velocity)
  x def1/1 -> Damper/1(displacement)
  Damper/1(F_d) -> Simulink-PS Converter1/1
  F damper/1 -> Mux1/3
  vu/1 -> Mux/4
  x def/1 -> Mux1/1
  Fs/1 -> Add/2, Fs2as/1
  Fu2au/1 -> Mux1/8
  vs/1 -> Mux/2
  xr/1 -> Mux1/6, Derivative/1
  Fs2as/1 -> Mux1/7
  Add/1 -> Fu2au/1
  xt def/1 -> Mux1/5
  Derivative/1 -> Simulink-PS Converter/1
  Fu/1 -> Add/1
  xs/1 -> Mux/1
  xu/1 -> Mux/3
  v def/1 -> Mux1/2
  Damper/2(current_log) -> Mux1/4
  connections:
  v def/LConn1 -- v def1/LConn1 -- Deflection sensor/RConn2
  Ideal Force Sensor/RConn2 -- Fs/LConn1
  Air Spring/LConn1 -- Deflection sensor/LConn1 -- Nonlinear Translational Spring/LConn1 -- Translational Hard Stop/LConn1 -- Ideal Force Sensor2/LConn1 -- Mu/RConn1 -- Ks/LConn1
  tire def sensor/RConn1 -- mu sensor/RConn1 -- Kt/RConn1 -- Ideal Force Sensor1/LConn1
  mu sensor/LConn1 -- Ideal Translational Velocity Source/LConn1 -- Mechanical Translational Reference/LConn1 -- Solver Configuration/RConn1 -- ms sensor/LConn1
  Ideal Force Sensor/RConn1 -- Ms/LConn1 -- ms sensor/RConn1
  Deflection sensor/RConn1 -- Ideal Force Source/RConn2 -- Ideal Force Sensor/LConn1 -- Ks/RConn1 -- Air Spring/RConn1 -- Translational Hard Stop/RConn1 -- Nonlinear Translational Spring/RConn1
  tire def sensor/LConn1 -- Kt/LConn1 -- Ideal Translational Velocity Source/RConn2
  xu/LConn1 -- mu sensor/RConn3
  Simulink-PS Converter/RConn1 -- Ideal Translational Velocity Source/RConn1
  x def/LConn1 -- x def1/LConn1 -- Deflection sensor/RConn3
  xs/LConn1 -- ms sensor/RConn3
  vs/LConn1 -- ms sensor/RConn2
  vu/LConn1 -- mu sensor/RConn2
  Ideal Force Sensor1/RConn2 -- Fu/LConn1
  tire def sensor/RConn3 -- xt def/LConn1
  Ideal Force Sensor1/RConn1 -- Mu/LConn1
  F damper/LConn1 -- Ideal Force Sensor2/RConn2
  Ideal Force Sensor2/RConn1 -- Ideal Force Source/LConn1
  Simulink-PS Converter1/RConn1 -- Ideal Force Source/RConn1

== system quarter_sus_imp/QuarterSuspension /Subsystem1/Semi Active Suspension ==
  act : Inport
  xr : Inport  Port=2
  Add{,2..4} (4 alike) : Sum  Inputs=+-
  Add1 : Sum
  Damper : Subsystem  Variant=on  VariantControlMode=label  VariantControl=Choice  LabelModeActiveChoice=Semi-active
  Divide : Product  Inputs=*/
  Divide1 : Product  Inputs=*/
  Gain : Gain  Gain=-1
  Mux : Mux
  Mux1 : Mux  Inputs=8
  ks : Gain  Gain=20000
  kt : Gain  Gain=200000
  ms : Constant  Value=400
  mu : Constant  Value=40
  vs0 : Integrator
  vu0 : Integrator
  xs0 : Integrator
  xu0 : Integrator
  state : Outport
  info : Outport  Port=2
  wires:
  Divide/1 -> Gain/1
  vu0/1 -> Mux/4, Add2/2, xu0/1  "vu"
  kt/1 -> Add/2
  xu0/1 -> Mux/3, Add3/2, Add4/1  "xu"
  xs0/1 -> Mux/1, Add3/1  "xs"
  ks/1 -> Add1/1
  Add1/1 -> Divide/1, Add/1
  xr/1 -> Mux1/6, Add4/2
  Add3/1 -> ks/1, Mux1/1, Damper/1(displacement)
  Add2/1 -> Damper/2(velocity), Mux1/2
  ms/1 -> Divide/2
  Damper/1(F_d) -> Mux1/3, Add1/2
  Add4/1 -> Mux1/5, kt/1
  mu/1 -> Divide1/2
  Damper/2(current_log) -> Mux1/4
  Gain/1 -> Mux1/7, vs0/1  "as"
  vs0/1 -> Mux/2, xs0/1, Add2/1  "vs"
  Divide1/1 -> Mux1/8, vu0/1  "au"
  act/1 -> Damper/3(current)
  Mux/1 -> state/1
  Mux1/1 -> info/1
  Add/1 -> Divide1/1

== system quarter_sus_imp/QuarterSuspension /Variant Subsystem/ADD ==
  state : Inport
  ref_info : Inport  Port=2
  train_action : Inport  Port=3
  Subsystem1 : Subsystem
  action : Outport
  wires:
  state/1 -> Subsystem1/1(state)
  Subsystem1/1(action) -> action/1

== system quarter_sus_imp/QuarterSuspension /Variant Subsystem/H1_power_min ==
  state : Inport
  ref_info : Inport  Port=2
  train_action : Inport  Port=3
  Subsystem1 : Subsystem
  action : Outport
  wires:
  Subsystem1/1(action) -> action/1
  state/1 -> Subsystem1/1(state)

== system quarter_sus_imp/QuarterSuspension /Variant Subsystem/IDA-PBC ==
  state : Inport
  ref_info : Inport  Port=2
  train_action : Inport  Port=3
  Subsystem : Subsystem  Variant=on  VariantControlMode=label  VariantControl=Choice  LabelModeActiveChoice=My_IDA_ISD
  action : Outport
  wires:
  state/1 -> Subsystem/1(In1)
  Subsystem/1(u) -> action/1

== system quarter_sus_imp/QuarterSuspension /Variant Subsystem/Openloop ==
  Open-loop input : Constant  Value=0.5
  action : Outport
  wires:
  Open-loop input/1 -> action/1

== system quarter_sus_imp/QuarterSuspension /Variant Subsystem/PDD ==
  state : Inport
  ref_info : Inport  Port=2
  train_action : Inport  Port=3
  Subsystem1 : Subsystem
  action : Outport
  wires:
  Subsystem1/1(action) -> action/1
  state/1 -> Subsystem1/1(state)

== system quarter_sus_imp/QuarterSuspension /Variant Subsystem/SH-ADD ==
  state : Inport
  ref_info : Inport  Port=2
  train_action : Inport  Port=3
  Subsystem1 : Subsystem
  action : Outport
  wires:
  Subsystem1/1(action) -> action/1
  state/1 -> Subsystem1/1(state)

== system quarter_sus_imp/QuarterSuspension /Variant Subsystem/Skyhook ==
  state : Inport
  ref_info : Inport  Port=2
  train_action : Inport  Port=3
  Subsystem : Subsystem
  Terminator : Terminator
  Terminator1 : Terminator
  action : Outport
  wires:
  train_action/1 -> Terminator/1
  ref_info/1 -> Terminator1/1
  state/1 -> Subsystem/1(In1)
  Subsystem/1(Out8) -> action/1

== system quarter_sus_imp/QuarterSuspension /Variant Subsystem/Train-Force ==
  train_action : Inport
  action : Outport
  wires:
  train_action/1 -> action/1

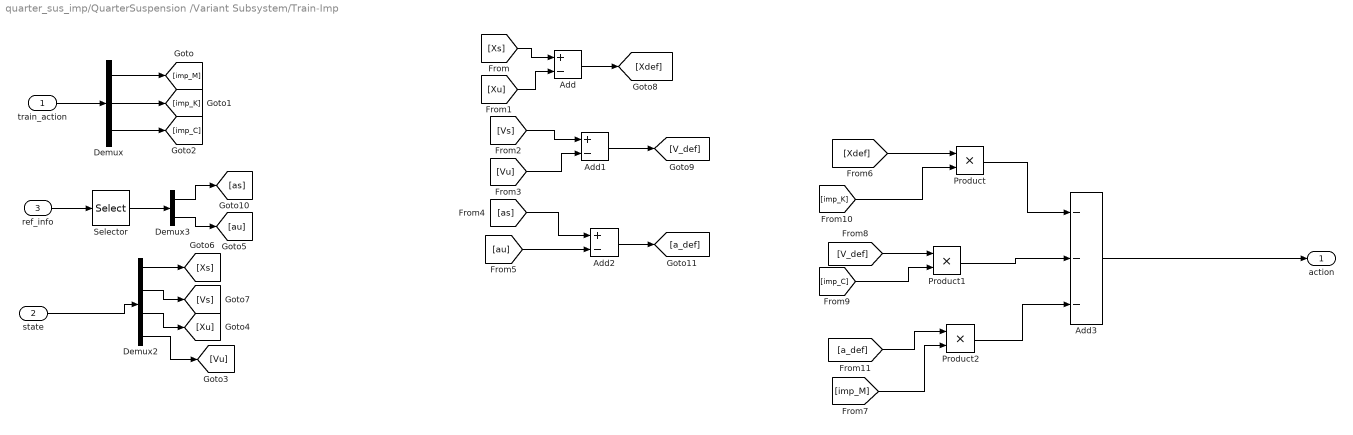
== system quarter_sus_imp/QuarterSuspension /Variant Subsystem/Train-Imp ==
  train_action : Inport  PortDimensions=3
  state : Inport  Port=2
  ref_info : Inport  Port=3
  Add : Sum  Inputs=+-
  Add1 : Sum  Inputs=+-
  Add2 : Sum  Inputs=+-
  Add3 : Sum  Inputs=---
  Demux : Demux  Outputs=3
  Demux2 : Demux
  Demux3 : Demux  Outputs=2
  Product : Product
  Product1 : Product
  Product2 : Product
  Selector : Selector  InputPortWidth=8  IndexOptions=Index vector (dialog)  Indices=[7 8]  OutputSizes=1
  action : Outport
  wires:
  Add3/1 -> action/1
  train_action/1 -> Demux/1
  Demux/2 -> [imp_K]
  Demux/1 -> [imp_M]
  Demux/3 -> [imp_C]
  Demux2/1 -> [Xs]
  Demux2/2 -> [Vs]
  Demux2/3 -> [Xu]
  Demux2/4 -> [Vu]
  state/1 -> Demux2/1
  ref_info/1 -> Selector/1
  Selector/1 -> Demux3/1
  Demux3/1 -> [as]
  Demux3/2 -> [au]
  [Xs] -> Add/1
  [Xu] -> Add/2
  Add/1 -> [Xdef]
  [Vs] -> Add1/1
  [Vu] -> Add1/2
  Add1/1 -> [V_def]
  [as] -> Add2/1
  [au] -> Add2/2
  Add2/1 -> [a_def]
  [Xdef] -> Product/1
  [imp_M] -> Product2/2
  [V_def] -> Product1/1
  [imp_C] -> Product1/2
  [imp_K] -> Product/2
  [a_def] -> Product2/1
  Product2/1 -> Add3/3
  Product1/1 -> Add3/2
  Product/1 -> Add3/1

== system quarter_sus_imp/QuarterSuspension /Variant Subsystem/Vaildation-3para-feedback ==
  state : Inport
  Demux1 : Demux  Outputs=11
  Impedance Controller : Subsystem
  Memory : Memory
  Mux1 : Mux  Inputs=5
  Rate Transition : RateTransition
  Rate Transition1 : RateTransition
  Subsystem : Subsystem  Variant=on  VariantControlMode=label  VariantControl=Choice  LabelModeActiveChoice=ONNX
  Terminator{1..5} (5 alike) : Terminator
  obsprocess : MATLAB Function  TreatAsAtomicUnit=on  SystemSampleTime=0.01
      settings: MinAlgLoopOccurrences=on
  action : Outport
  wires:
  Demux1/10 -> Terminator5/1
  Demux1/8 -> Mux1/4  "deflection"
  Rate Transition1/1 -> Impedance Controller/1(feedback_para)
  state/1 -> Memory/1
  Impedance Controller/1(F_imp) -> action/1
  Demux1/2 -> Mux1/2
  Demux1/6 -> Terminator3/1
  Mux1/1 -> Impedance Controller/2(est_state)
  Demux1/9 -> Mux1/5
  Demux1/7 -> Terminator4/1
  Demux1/5 -> Terminator2/1
  Demux1/1 -> Mux1/1
  Demux1/3 -> Mux1/3  "as"
  Demux1/4 -> Terminator1/1
  obsprocess/1(obs) -> Subsystem/1(In1)
  Memory/1 -> Rate Transition/1, Demux1/1
  Rate Transition/1 -> obsprocess/1(state)
  Subsystem/1(real_act) -> Rate Transition1/1

== system quarter_sus_imp/QuarterSuspension /Variant Subsystem/Vaildation-Force ==
  state : Inport
  Level-2 MATLAB S-Function : M-S-Function  FunctionName=gops_validation_bridge  Parameters='D:\Project\GOPS\transform_onnx_network\simu_quartersusconti\DDPG_231115-152105\network_DDPG_45050_opt.pt'
  Rate Transition : RateTransition
  Rate Transition1 : RateTransition
  obsprocess : MATLAB Function  TreatAsAtomicUnit=on  SystemSampleTime=0.01
      settings: MinAlgLoopOccurrences=on
  action : Outport
  wires:
  obsprocess/1(obs) -> Level-2 MATLAB S-Function/1
  state/1 -> Rate Transition/1
  Level-2 MATLAB S-Function/1 -> Rate Transition1/1
  Rate Transition/1 -> obsprocess/1(state)
  Rate Transition1/1 -> action/1

== system quarter_sus_imp/QuarterSuspension /Variant Subsystem/Vaildation-Imp ==
  state : Inport
  Constant : Constant  Value=imp_Ks
  Constant1 : Constant  Value=imp_Cs
  Constant2 : Constant  Value=imp_Ms
  Demux1 : Demux  Outputs=11
  Impedance Controller : Subsystem
  Level-2 MATLAB S-Function : M-S-Function  FunctionName=gops_validation_bridge  Parameters='D:\Project\GOPS\transform_onnx_network\simu_imp_quartersus\DDPG_231116-143445\network_DDPG_11500_opt.pt'
  Memory : Memory
  Memory1 : Memory
  Mux : Mux  Inputs=3
  Mux1 : Mux
  Rate Transition : RateTransition
  Rate Transition1 : RateTransition
  Terminator{,1..5} (6 alike) : Terminator
  actprocess : MATLAB Function  TreatAsAtomicUnit=on  SystemSampleTime=10
      settings: MinAlgLoopOccurrences=on
  obsprocess : MATLAB Function  TreatAsAtomicUnit=on  SystemSampleTime=10
      settings: MinAlgLoopOccurrences=on
  action : Outport
  wires:
  Constant1/1 -> Mux/3
  Mux1/1 -> Impedance Controller/3(est_state)
  Constant/1 -> Mux/2
  Memory1/1 -> Memory/1, Rate Transition/1
  Impedance Controller/1(F_imp) -> action/1
  state/1 -> Memory1/1
  obsprocess/1(obs) -> Level-2 MATLAB S-Function/1
  Rate Transition1/1 -> Impedance Controller/1(Imp_para)
  Demux1/5 -> Terminator2/1
  Demux1/8 -> Mux1/4  "deflection"
  Demux1/1 -> Mux1/1
  Demux1/7 -> Mux1/3
  Demux1/4 -> Terminator1/1
  Demux1/10 -> Terminator5/1
  Demux1/3 -> Terminator/1  "as"
  Level-2 MATLAB S-Function/1 -> actprocess/1(act)
  actprocess/1(real_act) -> Rate Transition1/1
  Mux/1 -> Impedance Controller/2(est_para)
  Demux1/6 -> Terminator3/1
  Rate Transition/1 -> obsprocess/1(state)
  Demux1/2 -> Mux1/2
  Memory/1 -> Demux1/1
  Demux1/9 -> Terminator4/1
  Constant2/1 -> Mux/1

== system quarter_sus_imp/QuarterSuspension /Variant Subsystem/impedance ==
  state : Inport
  Constant : Constant  Value=imp_Ks
  Constant1 : Constant  Value=imp_Cs
  Constant2 : Constant  Value=imp_Ms
  Demux1 : Demux  Outputs=11
  Impedance Controller1 : Subsystem
  Memory : Memory
  Mux : Mux  Inputs=3
  Mux1 : Mux
  Mux2 : Mux  Inputs=3
  Open-loop imp_C : Constant  Value=200
  Open-loop imp_K : Constant  Value=1000
  Open-loop imp_M : Constant  Value=375
  Terminator{,1..5} (6 alike) : Terminator
  action : Outport
  wires:
  Open-loop imp_M/1 -> Mux2/1
  Demux1/4 -> Terminator1/1
  Constant/1 -> Mux/2
  Demux1/3 -> Terminator/1  "as"
  state/1 -> Memory/1
  Mux2/1 -> Impedance Controller1/1(Imp_para)
  Demux1/7 -> Mux1/3
  Demux1/8 -> Mux1/4  "deflection"
  Demux1/6 -> Terminator3/1
  Memory/1 -> Demux1/1
  Demux1/1 -> Mux1/1
  Constant1/1 -> Mux/3
  Open-loop imp_C/1 -> Mux2/3
  Mux/1 -> Impedance Controller1/2(est_para)
  Demux1/10 -> Terminator5/1
  Mux1/1 -> Impedance Controller1/3(est_state)
  Demux1/2 -> Mux1/2
  Constant2/1 -> Mux/1
  Open-loop imp_K/1 -> Mux2/2
  Demux1/9 -> Terminator4/1
  Impedance Controller1/1(F_imp) -> action/1
  Demux1/5 -> Terminator2/1

== system quarter_sus_imp/QuarterSuspension /Variant Subsystem/train_IMP_force ==
  state : Inport
  ref_info : Inport  Port=2
  train_action : Inport  Port=3
  action : Outport
